simulink model "SF_simu"  (R2015a)
settings: Solver=ode45  StartTime=0.0  StopTime=10.0  RelTol=1e-3
values from neighbouring files (symbols this model uses):
  h1 = freqz(b1,a1,length(x64)/2)    [SF.m]    (also in SF2.m; SF3.m; SF_simulink.m = filt .* hamming(length(n))'; passeBasDownsample.m = filt .* hamming(length(n))')
  Osc = sin(2*pi*LO2*time)    [SF.m]    (also in SF2.m; SF_simulink.m = sin(2*pi*LO2*time)*2; passeBasDownsample.m = sin(2*pi*LO2*time)*2)
undefined symbols (not defined in the file or in its folder): a1, a2, b1, b2
libraries: dspstat3 x1
settings Model: Creator=Julien  LastModifiedBy=Julien

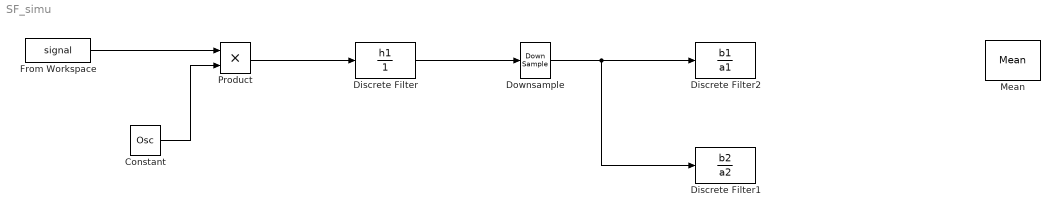
== system SF_simu ==
  Constant : Constant  Value=Osc
  Discrete Filter : DiscreteFilter  Numerator=h1  Denominator=1
  Discrete Filter1 : DiscreteFilter  Numerator=b2  Denominator=a2
  Discrete Filter2 : DiscreteFilter  Numerator=b1  Denominator=a1
  Downsample : DownSample  N=64  RateOptions=Allow multirate processing
  From Workspace : FromWorkspace  VariableName=signal  SampleTime=0
  Mean : dspstat3/Mean  run=off  reset_popup=None  InputProcessing=Columns as channels (frame based)  directionMode=Specified dimension  dimension=20  treatSBRowAsCol=off  roiEnable=off  roiType=Rectangles  roiPortion=Entire ROI  roiOutput=Individual statistics for each ROI  roiFlag=off  outputDataTypeStr=Inherit: Same as accumulator  outputLastDataTypeStr=Inherit: Same as accumulator  outputMin=[]  outputMax=[]  roundingMode=Floor  overflowMode=off
  Product : Product
  wires:
  From Workspace/1 -> Product/1
  Constant/1 -> Product/2
  Product/1 -> Discrete Filter/1
  Discrete Filter/1 -> Downsample/1
  Downsample/1 -> Discrete Filter1/1, Discrete Filter2/1
